simulink model "warplab_mimo_4x4"  (Simulink 6.6)
settings: Solver=ode45  StartTime=0.0  StopTime=50000  RelTol=1e-3
undefined symbols (not defined in the file): gcbh, xlBlockLoadCallback, xlGetSimulinkPeriod
libraries: xbsIndex_r4 x305, WARP_Blockset x16
(part 2 of 4)

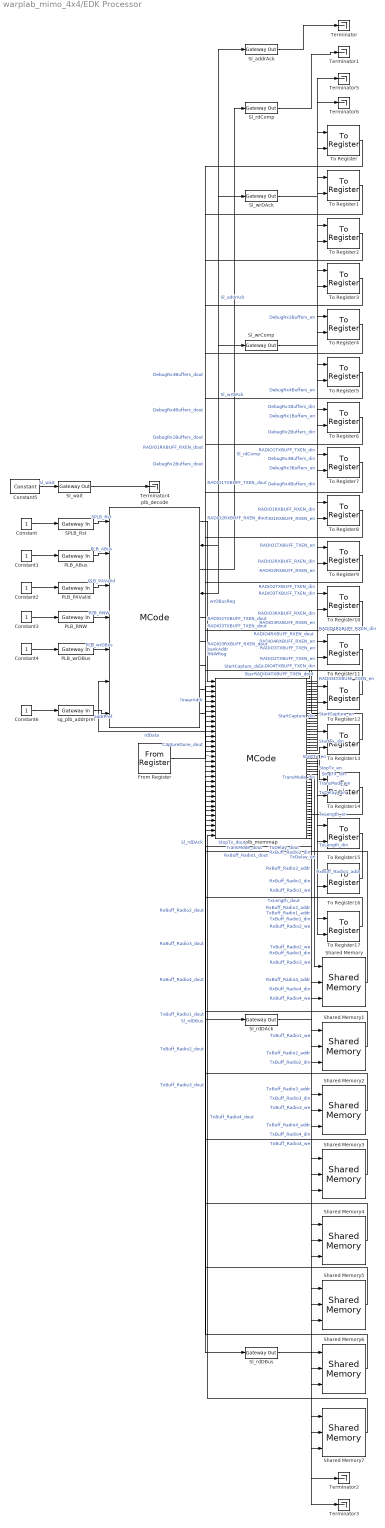
== system warplab_mimo_4x4/EDK Processor ==
  Constant{,1..4,6} (6 alike) : Constant
  Constant5 : xbsIndex_r4/Constant  arith_type=Unsigned  const=0  n_bits=1  bin_pt=0  explicit_period=on  period=xlGetSimulinkPeriod(gcb)  equ=P=C  opselect=C  inp2=PCIN>>17  opr=+  inp1=P  carry=CIN  dbl_ovrd=off  block_type=constant
  From Register : xbsIndex_r4/From Register  shared_memory_name='CaptureDone'  init=0  period=xlGetSimulinkPeriod(gcb)  ownership=Owned and initialized elsewhere  arith_type=Unsigned  n_bits=1  bin_pt=0  dbl_ovrd=off  block_type=fromreg
      settings: AttributesFormatString=<< %<shared_memory_name> >>  infoedit="Register block that reads data to a shared memory register.  Delay of one sample period."  block_version=10.1.3
  PLB_ABus : xbsIndex_r4/Gateway In  arith_type=Unsigned  n_bits=32  bin_pt=0  quantization="Round  (unbiased: +/- Inf)"  overflow=Saturate  period=xlGetSimulinkPeriod(gcb)  dbl_ovrd=off  timing_constraint=None  locs_specified=off  LOCs={}  block_type=gatewayin
      settings: infoedit="Gateway in block.  Converts inputs of type Simulink integer, double and fixed point to  Xilinx fixed point type.<P><P>Hardware notes:  In hardware these blocks become top level input ports."  sginterface={'Xilinx'=>{'jtaghwcosim'=>{'non_memory_mapped_port'=>'PLB_ABus'}},'iopad'=>{'constraint'=>'#'}}  block_version=10.1.3
  PLB_PAValid : xbsIndex_r4/Gateway In  arith_type=Unsigned  n_bits=1  bin_pt=0  quantization="Round  (unbiased: +/- Inf)"  overflow=Saturate  period=xlGetSimulinkPeriod(gcb)  dbl_ovrd=off  timing_constraint=None  locs_specified=off  LOCs={}  block_type=gatewayin
      settings: infoedit="Gateway in block.  Converts inputs of type Simulink integer, double and fixed point to  Xilinx fixed point type.<P><P>Hardware notes:  In hardware these blocks become top level input ports."  sginterface={'Xilinx'=>{'jtaghwcosim'=>{'non_memory_mapped_port'=>'PLB_PAValid'}},'iopad'=>{'constraint'=>'#'}}  block_version=10.1.3
  PLB_RNW : xbsIndex_r4/Gateway In  arith_type=Unsigned  n_bits=1  bin_pt=0  quantization="Round  (unbiased: +/- Inf)"  overflow=Saturate  period=xlGetSimulinkPeriod(gcb)  dbl_ovrd=off  timing_constraint=None  locs_specified=off  LOCs={}  block_type=gatewayin
      settings: infoedit="Gateway in block.  Converts inputs of type Simulink integer, double and fixed point to  Xilinx fixed point type.<P><P>Hardware notes:  In hardware these blocks become top level input ports."  sginterface={'Xilinx'=>{'jtaghwcosim'=>{'non_memory_mapped_port'=>'PLB_RNW'}},'iopad'=>{'constraint'=>'#'}}  block_version=10.1.3
  PLB_wrDBus : xbsIndex_r4/Gateway In  arith_type=Unsigned  n_bits=32  bin_pt=0  quantization="Round  (unbiased: +/- Inf)"  overflow=Saturate  period=xlGetSimulinkPeriod(gcb)  dbl_ovrd=off  timing_constraint=None  locs_specified=off  LOCs={}  block_type=gatewayin
      settings: infoedit="Gateway in block.  Converts inputs of type Simulink integer, double and fixed point to  Xilinx fixed point type.<P><P>Hardware notes:  In hardware these blocks become top level input ports."  sginterface={'Xilinx'=>{'jtaghwcosim'=>{'non_memory_mapped_port'=>'PLB_wrDBus'}},'iopad'=>{'constraint'=>'#'}}  block_version=10.1.3
  SPLB_Rst : xbsIndex_r4/Gateway In  arith_type=Unsigned  n_bits=1  bin_pt=0  quantization="Round  (unbiased: +/- Inf)"  overflow=Saturate  period=xlGetSimulinkPeriod(gcb)  dbl_ovrd=off  timing_constraint=None  locs_specified=off  LOCs={}  block_type=gatewayin
      settings: infoedit="Gateway in block.  Converts inputs of type Simulink integer, double and fixed point to  Xilinx fixed point type.<P><P>Hardware notes:  In hardware these blocks become top level input ports."  sginterface={'Xilinx'=>{'jtaghwcosim'=>{'non_memory_mapped_port'=>'SPLB_Rst'}},'iopad'=>{'constraint'=>'#'}}  block_version=10.1.3
  Shared Memory : xbsIndex_r4/Shared Memory  shared_memory_name='RxBuff_Radio1'  depth=16384  ownership=Owned and Initialized Elsewhere  initVector=sin(pi*(0:15)/16)  mutex=Unprotected  mode=Read and Write  write_mode=Read After Write  time_out=0  latency=1  explicit_data_type=off  arith_type=Unsigned  n_bits=32  bin_pt=0  implementation=Block RAM  use_rpm=off  block_type=shmem
      settings: AttributesFormatString=<< %<shared_memory_name> >>  block_version=10.1.3
  Shared Memory1 : xbsIndex_r4/Shared Memory  shared_memory_name='RxBuff_Radio2'  depth=16384  ownership=Owned and Initialized Elsewhere  initVector=sin(pi*(0:15)/16)  mutex=Unprotected  mode=Read and Write  write_mode=Read After Write  time_out=0  latency=1  explicit_data_type=off  arith_type=Unsigned  n_bits=32  bin_pt=0  implementation=Block RAM  use_rpm=off  block_type=shmem
      settings: AttributesFormatString=<< %<shared_memory_name> >>  block_version=10.1.3
  Shared Memory2 : xbsIndex_r4/Shared Memory  shared_memory_name='RxBuff_Radio3'  depth=16384  ownership=Owned and Initialized Elsewhere  initVector=sin(pi*(0:15)/16)  mutex=Unprotected  mode=Read and Write  write_mode=Read After Write  time_out=0  latency=1  explicit_data_type=off  arith_type=Unsigned  n_bits=32  bin_pt=0  implementation=Block RAM  use_rpm=off  block_type=shmem
      settings: AttributesFormatString=<< %<shared_memory_name> >>  block_version=10.1.3
  Shared Memory3 : xbsIndex_r4/Shared Memory  shared_memory_name='RxBuff_Radio4'  depth=16384  ownership=Owned and Initialized Elsewhere  initVector=sin(pi*(0:15)/16)  mutex=Unprotected  mode=Read and Write  write_mode=Read After Write  time_out=0  latency=1  explicit_data_type=off  arith_type=Unsigned  n_bits=32  bin_pt=0  implementation=Block RAM  use_rpm=off  block_type=shmem
      settings: AttributesFormatString=<< %<shared_memory_name> >>  block_version=10.1.3
  Shared Memory4 : xbsIndex_r4/Shared Memory  shared_memory_name='TxBuff_Radio1'  depth=16384  ownership=Owned and Initialized Elsewhere  initVector=sin(pi*(0:15)/16)  mutex=Unprotected  mode=Read and Write  write_mode=Read After Write  time_out=0  latency=1  explicit_data_type=off  arith_type=Unsigned  n_bits=32  bin_pt=0  implementation=Block RAM  use_rpm=off  block_type=shmem
      settings: AttributesFormatString=<< %<shared_memory_name> >>  block_version=10.1.3
  Shared Memory5 : xbsIndex_r4/Shared Memory  shared_memory_name='TxBuff_Radio2'  depth=16384  ownership=Owned and Initialized Elsewhere  initVector=sin(pi*(0:15)/16)  mutex=Unprotected  mode=Read and Write  write_mode=Read After Write  time_out=0  latency=1  explicit_data_type=off  arith_type=Unsigned  n_bits=32  bin_pt=0  implementation=Block RAM  use_rpm=off  block_type=shmem
      settings: AttributesFormatString=<< %<shared_memory_name> >>  block_version=10.1.3
  Shared Memory6 : xbsIndex_r4/Shared Memory  shared_memory_name='TxBuff_Radio3'  depth=16384  ownership=Owned and Initialized Elsewhere  initVector=sin(pi*(0:15)/16)  mutex=Unprotected  mode=Read and Write  write_mode=Read After Write  time_out=0  latency=1  explicit_data_type=off  arith_type=Unsigned  n_bits=32  bin_pt=0  implementation=Block RAM  use_rpm=off  block_type=shmem
      settings: AttributesFormatString=<< %<shared_memory_name> >>  block_version=10.1.3
  Shared Memory7 : xbsIndex_r4/Shared Memory  shared_memory_name='TxBuff_Radio4'  depth=16384  ownership=Owned and Initialized Elsewhere  initVector=sin(pi*(0:15)/16)  mutex=Unprotected  mode=Read and Write  write_mode=Read After Write  time_out=0  latency=1  explicit_data_type=off  arith_type=Unsigned  n_bits=32  bin_pt=0  implementation=Block RAM  use_rpm=off  block_type=shmem
      settings: AttributesFormatString=<< %<shared_memory_name> >>  block_version=10.1.3
  Sl_addrAck : xbsIndex_r4/Gateway Out  hdl_port=on  timing_constraint=None  locs_specified=off  LOCs={}  block_type=gatewayout
      settings: infoedit="Gateway out block.  Converts Xilinx fixed point inputs into ouputs of type Simulink integer, double, or fixed point.<P><P>Hardware notes:  In hardware these blocks become top level output ports or are discarded, depending on how they are configured."  sginterface={'Xilinx'=>{'jtaghwcosim'=>{'non_memory_mapped_port'=>'Sl_addrAck'}},'iopad'=>{'constraint'=>'#'}}  block_version=10.1.3
  Sl_rdComp : xbsIndex_r4/Gateway Out  hdl_port=on  timing_constraint=None  locs_specified=off  LOCs={}  block_type=gatewayout
      settings: infoedit="Gateway out block.  Converts Xilinx fixed point inputs into ouputs of type Simulink integer, double, or fixed point.<P><P>Hardware notes:  In hardware these blocks become top level output ports or are discarded, depending on how they are configured."  sginterface={'Xilinx'=>{'jtaghwcosim'=>{'non_memory_mapped_port'=>'Sl_rdComp'}},'iopad'=>{'constraint'=>'#'}}  block_version=10.1.3
  Sl_rdDAck : xbsIndex_r4/Gateway Out  hdl_port=on  timing_constraint=None  locs_specified=off  LOCs={}  block_type=gatewayout
      settings: infoedit="Gateway out block.  Converts Xilinx fixed point inputs into ouputs of type Simulink integer, double, or fixed point.<P><P>Hardware notes:  In hardware these blocks become top level output ports or are discarded, depending on how they are configured."  sginterface={'Xilinx'=>{'jtaghwcosim'=>{'non_memory_mapped_port'=>'Sl_rdDAck'}},'iopad'=>{'constraint'=>'#'}}  block_version=10.1.3
  Sl_rdDBus : xbsIndex_r4/Gateway Out  hdl_port=on  timing_constraint=None  locs_specified=off  LOCs={}  block_type=gatewayout
      settings: infoedit="Gateway out block.  Converts Xilinx fixed point inputs into ouputs of type Simulink integer, double, or fixed point.<P><P>Hardware notes:  In hardware these blocks become top level output ports or are discarded, depending on how they are configured."  sginterface={'Xilinx'=>{'jtaghwcosim'=>{'non_memory_mapped_port'=>'Sl_rdDBus'}},'iopad'=>{'constraint'=>'#'}}  block_version=10.1.3
  Sl_wait : xbsIndex_r4/Gateway Out  hdl_port=on  timing_constraint=None  locs_specified=off  LOCs={}  block_type=gatewayout
      settings: infoedit="Gateway out block.  Converts Xilinx fixed point inputs into ouputs of type Simulink integer, double, or fixed point.<P><P>Hardware notes:  In hardware these blocks become top level output ports or are discarded, depending on how they are configured."  sginterface={'Xilinx'=>{'jtaghwcosim'=>{'non_memory_mapped_port'=>'Sl_wait'}},'iopad'=>{'constraint'=>'#'}}  block_version=10.1.3
  Sl_wrComp : xbsIndex_r4/Gateway Out  hdl_port=on  timing_constraint=None  locs_specified=off  LOCs={}  block_type=gatewayout
      settings: infoedit="Gateway out block.  Converts Xilinx fixed point inputs into ouputs of type Simulink integer, double, or fixed point.<P><P>Hardware notes:  In hardware these blocks become top level output ports or are discarded, depending on how they are configured."  sginterface={'Xilinx'=>{'jtaghwcosim'=>{'non_memory_mapped_port'=>'Sl_wrComp'}},'iopad'=>{'constraint'=>'#'}}  block_version=10.1.3
  Sl_wrDAck : xbsIndex_r4/Gateway Out  hdl_port=on  timing_constraint=None  locs_specified=off  LOCs={}  block_type=gatewayout
      settings: infoedit="Gateway out block.  Converts Xilinx fixed point inputs into ouputs of type Simulink integer, double, or fixed point.<P><P>Hardware notes:  In hardware these blocks become top level output ports or are discarded, depending on how they are configured."  sginterface={'Xilinx'=>{'jtaghwcosim'=>{'non_memory_mapped_port'=>'Sl_wrDAck'}},'iopad'=>{'constraint'=>'#'}}  block_version=10.1.3
  Terminator{,1..6} (7 alike) : Terminator
  To Register : xbsIndex_r4/To Register  shared_memory_name='DebugRx1Buffers'  init=0  ownership=Owned and initialized elsewhere  explicit_data_type=on  arith_type=Unsigned  n_bits=1  bin_pt=0  dbl_ovrd=off  block_type=toreg
      settings: AttributesFormatString=<< %<shared_memory_name> >>  infoedit="Register block that writes data to a shared memory register.  Delay of one sample period."  block_version=10.1.3
  To Register1 : xbsIndex_r4/To Register  shared_memory_name='DebugRx2Buffers'  init=0  ownership=Owned and initialized elsewhere  explicit_data_type=on  arith_type=Unsigned  n_bits=1  bin_pt=0  dbl_ovrd=off  block_type=toreg
      settings: AttributesFormatString=<< %<shared_memory_name> >>  infoedit="Register block that writes data to a shared memory register.  Delay of one sample period."  block_version=10.1.3
  To Register10 : xbsIndex_r4/To Register  shared_memory_name='RADIO4RXBUFF_RXEN'  init=0  ownership=Owned and initialized elsewhere  explicit_data_type=on  arith_type=Unsigned  n_bits=1  bin_pt=0  dbl_ovrd=off  block_type=toreg
      settings: AttributesFormatString=<< %<shared_memory_name> >>  infoedit="Register block that writes data to a shared memory register.  Delay of one sample period."  block_version=10.1.3
  To Register11 : xbsIndex_r4/To Register  shared_memory_name='RADIO4TXBUFF_TXEN'  init=0  ownership=Owned and initialized elsewhere  explicit_data_type=on  arith_type=Unsigned  n_bits=1  bin_pt=0  dbl_ovrd=off  block_type=toreg
      settings: AttributesFormatString=<< %<shared_memory_name> >>  infoedit="Register block that writes data to a shared memory register.  Delay of one sample period."  block_version=10.1.3
  To Register12 : xbsIndex_r4/To Register  shared_memory_name='StartCapture'  init=0  ownership=Owned and initialized elsewhere  explicit_data_type=on  arith_type=Unsigned  n_bits=1  bin_pt=0  dbl_ovrd=off  block_type=toreg
      settings: AttributesFormatString=<< %<shared_memory_name> >>  infoedit="Register block that writes data to a shared memory register.  Delay of one sample period."  block_version=10.1.3
  To Register13 : xbsIndex_r4/To Register  shared_memory_name='StartTx'  init=0  ownership=Owned and initialized elsewhere  explicit_data_type=on  arith_type=Unsigned  n_bits=1  bin_pt=0  dbl_ovrd=off  block_type=toreg
      settings: AttributesFormatString=<< %<shared_memory_name> >>  infoedit="Register block that writes data to a shared memory register.  Delay of one sample period."  block_version=10.1.3
  To Register14 : xbsIndex_r4/To Register  shared_memory_name='StopTx'  init=0  ownership=Owned and initialized elsewhere  explicit_data_type=on  arith_type=Unsigned  n_bits=1  bin_pt=0  dbl_ovrd=off  block_type=toreg
      settings: AttributesFormatString=<< %<shared_memory_name> >>  infoedit="Register block that writes data to a shared memory register.  Delay of one sample period."  block_version=10.1.3
  To Register15 : xbsIndex_r4/To Register  shared_memory_name='TransMode'  init=0  ownership=Owned and initialized elsewhere  explicit_data_type=on  arith_type=Unsigned  n_bits=1  bin_pt=0  dbl_ovrd=off  block_type=toreg
      settings: AttributesFormatString=<< %<shared_memory_name> >>  infoedit="Register block that writes data to a shared memory register.  Delay of one sample period."  block_version=10.1.3
  To Register16 : xbsIndex_r4/To Register  shared_memory_name='TxDelay'  init=0  ownership=Owned and initialized elsewhere  explicit_data_type=on  arith_type=Unsigned  n_bits=14  bin_pt=0  dbl_ovrd=off  block_type=toreg
      settings: AttributesFormatString=<< %<shared_memory_name> >>  infoedit="Register block that writes data to a shared memory register.  Delay of one sample period."  block_version=10.1.3
  To Register17 : xbsIndex_r4/To Register  shared_memory_name='TxLength'  init=0  ownership=Owned and initialized elsewhere  explicit_data_type=on  arith_type=Unsigned  n_bits=14  bin_pt=0  dbl_ovrd=off  block_type=toreg
      settings: AttributesFormatString=<< %<shared_memory_name> >>  infoedit="Register block that writes data to a shared memory register.  Delay of one sample period."  block_version=10.1.3
  To Register2 : xbsIndex_r4/To Register  shared_memory_name='DebugRx3Buffers'  init=0  ownership=Owned and initialized elsewhere  explicit_data_type=on  arith_type=Unsigned  n_bits=1  bin_pt=0  dbl_ovrd=off  block_type=toreg
      settings: AttributesFormatString=<< %<shared_memory_name> >>  infoedit="Register block that writes data to a shared memory register.  Delay of one sample period."  block_version=10.1.3
  To Register3 : xbsIndex_r4/To Register  shared_memory_name='DebugRx4Buffers'  init=0  ownership=Owned and initialized elsewhere  explicit_data_type=on  arith_type=Unsigned  n_bits=1  bin_pt=0  dbl_ovrd=off  block_type=toreg
      settings: AttributesFormatString=<< %<shared_memory_name> >>  infoedit="Register block that writes data to a shared memory register.  Delay of one sample period."  block_version=10.1.3
  To Register4 : xbsIndex_r4/To Register  shared_memory_name='RADIO1RXBUFF_RXEN'  init=0  ownership=Owned and initialized elsewhere  explicit_data_type=on  arith_type=Unsigned  n_bits=1  bin_pt=0  dbl_ovrd=off  block_type=toreg
      settings: AttributesFormatString=<< %<shared_memory_name> >>  infoedit="Register block that writes data to a shared memory register.  Delay of one sample period."  block_version=10.1.3
  To Register5 : xbsIndex_r4/To Register  shared_memory_name='RADIO1TXBUFF_TXEN'  init=0  ownership=Owned and initialized elsewhere  explicit_data_type=on  arith_type=Unsigned  n_bits=1  bin_pt=0  dbl_ovrd=off  block_type=toreg
      settings: AttributesFormatString=<< %<shared_memory_name> >>  infoedit="Register block that writes data to a shared memory register.  Delay of one sample period."  block_version=10.1.3
  To Register6 : xbsIndex_r4/To Register  shared_memory_name='RADIO2RXBUFF_RXEN'  init=0  ownership=Owned and initialized elsewhere  explicit_data_type=on  arith_type=Unsigned  n_bits=1  bin_pt=0  dbl_ovrd=off  block_type=toreg
      settings: AttributesFormatString=<< %<shared_memory_name> >>  infoedit="Register block that writes data to a shared memory register.  Delay of one sample period."  block_version=10.1.3
  To Register7 : xbsIndex_r4/To Register  shared_memory_name='RADIO2TXBUFF_TXEN'  init=0  ownership=Owned and initialized elsewhere  explicit_data_type=on  arith_type=Unsigned  n_bits=1  bin_pt=0  dbl_ovrd=off  block_type=toreg
      settings: AttributesFormatString=<< %<shared_memory_name> >>  infoedit="Register block that writes data to a shared memory register.  Delay of one sample period."  block_version=10.1.3
  To Register8 : xbsIndex_r4/To Register  shared_memory_name='RADIO3RXBUFF_RXEN'  init=0  ownership=Owned and initialized elsewhere  explicit_data_type=on  arith_type=Unsigned  n_bits=1  bin_pt=0  dbl_ovrd=off  block_type=toreg
      settings: AttributesFormatString=<< %<shared_memory_name> >>  infoedit="Register block that writes data to a shared memory register.  Delay of one sample period."  block_version=10.1.3
  To Register9 : xbsIndex_r4/To Register  shared_memory_name='RADIO3TXBUFF_TXEN'  init=0  ownership=Owned and initialized elsewhere  explicit_data_type=on  arith_type=Unsigned  n_bits=1  bin_pt=0  dbl_ovrd=off  block_type=toreg
      settings: AttributesFormatString=<< %<shared_memory_name> >>  infoedit="Register block that writes data to a shared memory register.  Delay of one sample period."  block_version=10.1.3
  plb_decode : xbsIndex_r4/MCode  mfname=xlmax  explicit_period=off  period=1  dbl_ovrd=off  enable_stdout=off  enable_debug=off  mfilecontent=|  suppress_output=1  defparams={}  hide_port_list={}  block_type=mcode
      | function [wrDBusReg, addrAck, rdComp, wrDAck, bankAddr, RNWReg, rdDAck, rdDBus, linearAddr] = ...
      |     plb_bus_decode(plbRst, plbABus, plbPAValid, plbRNW, plbWrDBus, rdData, addrPref)
      | 
      | % constant variables (TODO: should pass from outside)
      | ADDRPREF_LEN = 11;
      | BANKADDR_LEN = 2;
      | LINEARADDR_LEN = 17;
      | ABUS_LEN = 32;
      | DBUS_LEN = 32;
      | 
      | % declare and initialize persistent variables
      | % register input bus signals
      | persistent plbRstReg_, plbRstReg_ = xl_state(0, {xlBoolean});
      | persistent plbABusReg_, plbABusReg_ = xl_state(0, {xlUnsigned, ABUS_LEN, 0});
      | persistent plbPAValidReg_, plbPAValidReg_ = xl_state(0, {xlBoolean});
      | persistent plbRNWReg_, plbRNWReg_ = xl_state(0, {xlUnsigned, 1, 0});
      | persistent plbWrDBusReg_, plbWrDBusReg_ = xl_state(0, {xlUnsigned, DBUS_LEN, 0});
      | 
      | % ===== rest of the outputs =====
      | 
      | bankAddr   = xl_slice(plbABusReg_, 2+BANKADDR_LEN+LINEARADDR_LEN-1, 2+LINEARADDR_LEN);
      | linearAddr = xl_slice(plbABusReg_, 2+LINEARADDR_LEN-1, 2);
      | RNWReg = plbRNWReg_;
      | wrDBusReg = plbWrDBusReg_;
      | 
      | % ===== p_select =====
      | 
      | % register PAValid
      | persistent aValidReg, aValidReg = xl_state(0, {xlBoolean});
      | aValidReg = plbPAValidReg_;
      | 
      | % extract and register the address prefix
      | addrPref_in = xl_slice(plbABusReg_, xl_nbits(plbABusReg_)-1, xl_nbits(plbABusReg_)-ADDRPREF_LEN);
      | if addrPref_in == addrPref
      |     ps1 = true;
      | else 
      |     ps1 = false;
      | end 
      | 
      | persistent ps1Reg, ps1Reg = xl_state(0, ps1);
      | ps1Reg = ps1;
      | 
      | ps = xl_and(ps1Reg, aValidReg);
      | 
      | % ===== addrAck =====
      | 
      | % register ps
      | persistent psReg, psReg = xl_state(0, ps);
      | 
      | addrAck = xfix({xlUnsigned, 1, 0}, xl_and(xl_not(plbRstReg_), ps, xl_not(psReg)));
      | 
      | psReg = ps;
      | 
      | % ===== rdComp, rd/wr DAck =====
      |  
      | rdComp1 = xfix({xlUnsigned, 1, 0}, xl_and(addrAck, RNWReg));
      | 
      | NUM_rdCompDelay = 3;
      | persistent rdCompDelay, rdCompDelay = xl_state(zeros(1, NUM_rdCompDelay), rdComp1, NUM_rdCompDelay);
      | rdComp2 = rdCompDelay.back;
      | rdCompDelay.push_front_pop_back(rdComp1);
      | 
      | persistent rdCompReg, rdCompReg = xl_state(0, rdComp1);
      | rdComp = rdCompReg;
      | rdCompReg = rdComp2;
      | 
      | persistent rdDAckReg, rdDAckReg = xl_state(0, rdComp1);
      | rdDAck = rdDAckReg;
      | rdDAckReg = rdComp;
      | 
      | persistent wrDAckReg, wrDAckReg = xl_state(0, addrAck);
      | wrDAck = wrDAckReg;
      | wrDAckReg = xl_and(addrAck, xl_not(RNWReg));
      | 
      | % ===== rdDBus =====
      | 
      | rdSel = xl_or(rdComp2, rdComp);
      | 
      | if rdSel == 1
      |     rdDBus1 = rdData;
      | else
      |     rdDBus1 = 0;
      | end % if
      | 
      | persistent rdDBusReg, rdDBusReg = xl_state(0, rdDBus1);
      | rdDBus = rdDBusReg;
      | rdDBusReg = rdDBus1;
      | 
      | % rdDBus = xl_concat(rdDBus32, rdDBus32);
      | % rdDBus = rdDBus32;
      | 
      | % ===== update the persistent variables =====
      | 
      | plbRstReg_ = plbRst;
      | plbABusReg_ = plbABus;
      | plbPAValidReg_ = plbPAValid;
      | plbRNWReg_ = plbRNW;
      | plbWrDBusReg_ = xl_slice(plbWrDBus, DBUS_LEN-1, 0);
      settings: block_version=10.1.3
  plb_memmap : xbsIndex_r4/MCode  mfname=xlmax  explicit_period=off  period=1  dbl_ovrd=off  enable_stdout=off  enable_debug=off  mfilecontent=|  suppress_output=1  defparams={}  hide_port_list={}  block_type=mcode
      | function [read_bank_out, sm_DebugRx1Buffers_din, sm_DebugRx1Buffers_en, sm_DebugRx2Buffers_din, sm_DebugRx2Buffers_en, sm_DebugRx3Buffers_din, sm_DebugRx3Buffers_en, sm_DebugRx4Buffers_din, sm_DebugRx4Buffers_en, sm_RADIO1RXBUFF_RXEN_din, sm_RADIO1RXBUFF_RXEN_en, sm_RADIO1TXBUFF_TXEN_din, sm_RADIO1TXBUFF_TXEN_en, sm_RADIO2RXBUFF_RXEN_din, sm_RADIO2RXBUFF_RXEN_en, sm_RADIO2TXBUFF_TXEN_din, sm_RADIO2TXBUFF_TXEN_en, sm_RADIO3RXBUFF_RXEN_din, sm_RADIO3RXBUFF_RXEN_en, sm_RADIO3TXBUFF_TXEN_din, sm_RADIO3TXBUFF_TXEN_en, sm_RADIO4RXBUFF_RXEN_din, sm_RADIO4RXBUFF_RXEN_en, sm_RADIO4TXBUFF_TXEN_din, sm_RADIO4TXBUFF_TXEN_en, sm_StartCapture_din, sm_StartCapture_en, sm_StartTx_din, sm_StartTx_en, sm_StopTx_din, sm_StopTx_en, sm_TransMode_din, sm_TransMode_en, sm_TxDelay_din, sm_TxDelay_en, sm_TxLength_din, sm_TxLength_en, sm_RxBuff_Radio1_addr, sm_RxBuff_Radio1_din, sm_RxBuff_Radio1_we, sm_RxBuff_Radio2_addr, sm_RxBuff_Radio2_din, sm_RxBuff_Radio2_we, sm_RxBuff_Radio3_addr, sm_RxBuff_Radio3_din, sm_RxBuff_Radio3_we, sm_RxBuff_Radio4_addr, sm_RxBuff_Radio4_din, sm_RxBuff_Radio4_we, sm_TxBuff_Radio1_addr, sm_TxBuff_Radio1_din, sm_TxBuff_Radio1_we, sm_TxBuff_Radio2_addr, sm_TxBuff_Radio2_din, sm_TxBuff_Radio2_we, sm_TxBuff_Radio3_addr, sm_TxBuff_Radio3_din, sm_TxBuff_Radio3_we, sm_TxBuff_Radio4_addr, sm_TxBuff_Radio4_din, sm_TxBuff_Radio4_we] = plb_memmap(wrDBus, bankAddr, linearAddr, RNWReg, addrAck, sm_CaptureDone, sm_DebugRx1Buffers, sm_DebugRx2Buffers, sm_DebugRx3Buffers, sm_DebugRx4Buffers, sm_RADIO1RXBUFF_RXEN, sm_RADIO1TXBUFF_TXEN, sm_RADIO2RXBUFF_RXEN, sm_RADIO2TXBUFF_TXEN, sm_RADIO3RXBUFF_RXEN, sm_RADIO3TXBUFF_TXEN, sm_RADIO4RXBUFF_RXEN, sm_RADIO4TXBUFF_TXEN, sm_StartCapture, sm_StartTx, sm_StopTx, sm_TransMode, sm_TxDelay, sm_TxLength, sm_RxBuff_Radio1, sm_RxBuff_Radio2, sm_RxBuff_Radio3, sm_RxBuff_Radio4, sm_TxBuff_Radio1, sm_TxBuff_Radio2, sm_TxBuff_Radio3, sm_TxBuff_Radio4)
      | 
      | 
      | % connvert the input data to UFix_32_0 (the bus data type)
      | % 'From Register' blocks
      | % sm_CaptureDone_bus = xfix({xlUnsigned, 32, 0}, 0);
      | sm_CaptureDone_bus = xl_force(sm_CaptureDone, xlUnsigned, 0);
      | 
      | % 'To Register' blocks
      | 
      | % sm_DebugRx1Buffers_dout = xfix({xlUnsigned, 32, 0}, 0);
      | sm_DebugRx1Buffers_dout = xl_force(sm_DebugRx1Buffers, xlUnsigned, 0);
      | 
      | % sm_DebugRx2Buffers_dout = xfix({xlUnsigned, 32, 0}, 0);
      | sm_DebugRx2Buffers_dout = xl_force(sm_DebugRx2Buffers, xlUnsigned, 0);
      | 
      | % sm_DebugRx3Buffers_dout = xfix({xlUnsigned, 32, 0}, 0);
      | sm_DebugRx3Buffers_dout = xl_force(sm_DebugRx3Buffers, xlUnsigned, 0);
      | 
      | % sm_DebugRx4Buffers_dout = xfix({xlUnsigned, 32, 0}, 0);
      | sm_DebugRx4Buffers_dout = xl_force(sm_DebugRx4Buffers, xlUnsigned, 0);
      | 
      | % sm_RADIO1RXBUFF_RXEN_dout = xfix({xlUnsigned, 32, 0}, 0);
      | sm_RADIO1RXBUFF_RXEN_dout = xl_force(sm_RADIO1RXBUFF_RXEN, xlUnsigned, 0);
      | 
      | % sm_RADIO1TXBUFF_TXEN_dout = xfix({xlUnsigned, 32, 0}, 0);
      | sm_RADIO1TXBUFF_TXEN_dout = xl_force(sm_RADIO1TXBUFF_TXEN, xlUnsigned, 0);
      | 
      | % sm_RADIO2RXBUFF_RXEN_dout = xfix({xlUnsigned, 32, 0}, 0);
      | sm_RADIO2RXBUFF_RXEN_dout = xl_force(sm_RADIO2RXBUFF_RXEN, xlUnsigned, 0);
      | 
      | % sm_RADIO2TXBUFF_TXEN_dout = xfix({xlUnsigned, 32, 0}, 0);
      | sm_RADIO2TXBUFF_TXEN_dout = xl_force(sm_RADIO2TXBUFF_TXEN, xlUnsigned, 0);
      | 
      | % sm_RADIO3RXBUFF_RXEN_dout = xfix({xlUnsigned, 32, 0}, 0);
      | sm_RADIO3RXBUFF_RXEN_dout = xl_force(sm_RADIO3RXBUFF_RXEN, xlUnsigned, 0);
      | 
      | % sm_RADIO3TXBUFF_TXEN_dout = xfix({xlUnsigned, 32, 0}, 0);
      | sm_RADIO3TXBUFF_TXEN_dout = xl_force(sm_RADIO3TXBUFF_TXEN, xlUnsigned, 0);
      | 
      | % sm_RADIO4RXBUFF_RXEN_dout = xfix({xlUnsigned, 32, 0}, 0);
      | sm_RADIO4RXBUFF_RXEN_dout = xl_force(sm_RADIO4RXBUFF_RXEN, xlUnsigned, 0);
      | 
      | % sm_RADIO4TXBUFF_TXEN_dout = xfix({xlUnsigned, 32, 0}, 0);
      | sm_RADIO4TXBUFF_TXEN_dout = xl_force(sm_RADIO4TXBUFF_TXEN, xlUnsigned, 0);
      | 
      | % sm_StartCapture_dout = xfix({xlUnsigned, 32, 0}, 0);
      | sm_StartCapture_dout = xl_force(sm_StartCapture, xlUnsigned, 0);
      | 
      | % sm_StartTx_dout = xfix({xlUnsigned, 32, 0}, 0);
      | sm_StartTx_dout = xl_force(sm_StartTx, xlUnsigned, 0);
      | 
      | % sm_StopTx_dout = xfix({xlUnsigned, 32, 0}, 0);
      | sm_StopTx_dout = xl_force(sm_StopTx, xlUnsigned, 0);
      | 
      | % sm_TransMode_dout = xfix({xlUnsigned, 32, 0}, 0);
      | sm_TransMode_dout = xl_force(sm_TransMode, xlUnsigned, 0);
      | 
      | % sm_TxDelay_dout = xfix({xlUnsigned, 32, 0}, 0);
      | sm_TxDelay_dout = xl_force(sm_TxDelay, xlUnsigned, 0);
      | 
      | % sm_TxLength_dout = xfix({xlUnsigned, 32, 0}, 0);
      | sm_TxLength_dout = xl_force(sm_TxLength, xlUnsigned, 0);
      | 
      | 
      | % 'From FIFO' blocks
      | % 'To FIFO' blocks
      | % 'Shared Memory' blocks
      | % RxBuff_Radio1_bus = xfix({xlUnsigned, 32, 0}, 0);
      | sm_RxBuff_Radio1_bus = xl_force(sm_RxBuff_Radio1, xlUnsigned, 0);
      | 
      | % RxBuff_Radio2_bus = xfix({xlUnsigned, 32, 0}, 0);
      | sm_RxBuff_Radio2_bus = xl_force(sm_RxBuff_Radio2, xlUnsigned, 0);
      | 
      | % RxBuff_Radio3_bus = xfix({xlUnsigned, 32, 0}, 0);
      | sm_RxBuff_Radio3_bus = xl_force(sm_RxBuff_Radio3, xlUnsigned, 0);
      | 
      | % RxBuff_Radio4_bus = xfix({xlUnsigned, 32, 0}, 0);
      | sm_RxBuff_Radio4_bus = xl_force(sm_RxBuff_Radio4, xlUnsigned, 0);
      | 
      | % TxBuff_Radio1_bus = xfix({xlUnsigned, 32, 0}, 0);
      | sm_TxBuff_Radio1_bus = xl_force(sm_TxBuff_Radio1, xlUnsigned, 0);
      | 
      | % TxBuff_Radio2_bus = xfix({xlUnsigned, 32, 0}, 0);
      | sm_TxBuff_Radio2_bus = xl_force(sm_TxBuff_Radio2, xlUnsigned, 0);
      | 
      | % TxBuff_Radio3_bus = xfix({xlUnsigned, 32, 0}, 0);
      | sm_TxBuff_Radio3_bus = xl_force(sm_TxBuff_Radio3, xlUnsigned, 0);
      | 
      | % TxBuff_Radio4_bus = xfix({xlUnsigned, 32, 0}, 0);
      | sm_TxBuff_Radio4_bus = xl_force(sm_TxBuff_Radio4, xlUnsigned, 0);
      | 
      | 
      | % 'dout' ports of 'From Register' blocks
      | 
      | % registered register mux output
      | persistent reg_bank_out_reg; reg_bank_out_reg = xl_state(0, {xlUnsigned, 32, 0});
      | reg_bank_out = reg_bank_out_reg;
      | 
      | if linearAddr == 18
      |     reg_bank_out_reg = sm_CaptureDone_bus;
      | elseif linearAddr == 0
      |     reg_bank_out_reg = sm_DebugRx1Buffers_dout;
      | elseif linearAddr == 1
      |     reg_bank_out_reg = sm_DebugRx2Buffers_dout;
      | elseif linearAddr == 2
      |     reg_bank_out_reg = sm_DebugRx3Buffers_dout;
      | elseif linearAddr == 3
      |     reg_bank_out_reg = sm_DebugRx4Buffers_dout;
      | elseif linearAddr == 4
      |     reg_bank_out_reg = sm_RADIO1RXBUFF_RXEN_dout;
      | elseif linearAddr == 5
      |     reg_bank_out_reg = sm_RADIO1TXBUFF_TXEN_dout;
      | elseif linearAddr == 6
      |     reg_bank_out_reg = sm_RADIO2RXBUFF_RXEN_dout;
      | elseif linearAddr == 7
      |     reg_bank_out_reg = sm_RADIO2TXBUFF_TXEN_dout;
      | elseif linearAddr == 8
      |     reg_bank_out_reg = sm_RADIO3RXBUFF_RXEN_dout;
      | elseif linearAddr == 9
      |     reg_bank_out_reg = sm_RADIO3TXBUFF_TXEN_dout;
      | elseif linearAddr == 10
      |     reg_bank_out_reg = sm_RADIO4RXBUFF_RXEN_dout;
      | elseif linearAddr == 11
      |     reg_bank_out_reg = sm_RADIO4TXBUFF_TXEN_dout;
      | elseif linearAddr == 12
      |     reg_bank_out_reg = sm_StartCapture_dout;
      | elseif linearAddr == 13
      |     reg_bank_out_reg = sm_StartTx_dout;
      | elseif linearAddr == 14
      |     reg_bank_out_reg = sm_StopTx_dout;
      | elseif linearAddr == 15
      |     reg_bank_out_reg = sm_TransMode_dout;
      | elseif linearAddr == 16
      |     reg_bank_out_reg = sm_TxDelay_dout;
      | elseif linearAddr == 17
      |     reg_bank_out_reg = sm_TxLength_dout;
      | 
      | end
      | 
      | 
      | % 'From FIFO' and 'To FIFO' blocks
      | 
      | 
      | 
      | 
      | 
      | opCode = xl_concat(addrAck, RNWReg, bankAddr, linearAddr);
      | 
      | % 'Shared Memory' blocks
      | 
      | sm_RxBuff_Radio1_sel_value = xl_concat(xl_slice(linearAddr, ...
      |                                         xl_nbits(linearAddr) - 1, ...
      |                                         14) ...
      |                                     );
      | if sm_RxBuff_Radio1_sel_value == xfix({xlUnsigned, ...
      |                                         xl_nbits(linearAddr) - 14, ...
      |                                         0}, ...
      |                                         0);
      |     sm_RxBuff_Radio1_sel = true;
      | else
      |     sm_RxBuff_Radio1_sel = false;
      | end
      | sm_RxBuff_Radio2_sel_value = xl_concat(xl_slice(linearAddr, ...
      |                                         xl_nbits(linearAddr) - 1, ...
      |                                         14) ...
      |                                     );
      | if sm_RxBuff_Radio2_sel_value == xfix({xlUnsigned, ...
      |                                         xl_nbits(linearAddr) - 14, ...
      |                                         0}, ...
      |                                         1);
      |     sm_RxBuff_Radio2_sel = true;
      | else
      |     sm_RxBuff_Radio2_sel = false;
      | end
      | sm_RxBuff_Radio3_sel_value = xl_concat(xl_slice(linearAddr, ...
      |                                         xl_nbits(linearAddr) - 1, ...
      |                                         14) ...
      |                                     );
      | if sm_RxBuff_Radio3_sel_value == xfix({xlUnsigned, ...
      |                                         xl_nbits(linearAddr) - 14, ...
      |                                         0}, ...
      |                                         2);
      |     sm_RxBuff_Radio3_sel = true;
      | else
      |     sm_RxBuff_Radio3_sel = false;
      | end
      | sm_RxBuff_Radio4_sel_value = xl_concat(xl_slice(linearAddr, ...
      |                                         xl_nbits(linearAddr) - 1, ...
      |                                         14) ...
      |                                     );
      | if sm_RxBuff_Radio4_sel_value == xfix({xlUnsigned, ...
      |                                         xl_nbits(linearAddr) - 14, ...
      |                                         0}, ...
      |                                         3);
      |     sm_RxBuff_Radio4_sel = true;
      | else
      |     sm_RxBuff_Radio4_sel = false;
      | end
      | sm_TxBuff_Radio1_sel_value = xl_concat(xl_slice(linearAddr, ...
      |                                         xl_nbits(linearAddr) - 1, ...
      |                                         14) ...
      |                                     );
      | if sm_TxBuff_Radio1_sel_value == xfix({xlUnsigned, ...
      |                                         xl_nbits(linearAddr) - 14, ...
      |                                         0}, ...
      |                                         4);
      |     sm_TxBuff_Radio1_sel = true;
      | else
      |     sm_TxBuff_Radio1_sel = false;
      | end
      | sm_TxBuff_Radio2_sel_value = xl_concat(xl_slice(linearAddr, ...
      |                                         xl_nbits(linearAddr) - 1, ...
      |                                         14) ...
      |                                     );
      | if sm_TxBuff_Radio2_sel_value == xfix({xlUnsigned, ...
      |                                         xl_nbits(linearAddr) - 14, ...
      |                                         0}, ...
      |                                         5);
      |     sm_TxBuff_Radio2_sel = true;
      | else
      |     sm_TxBuff_Radio2_sel = false;
      | end
      | sm_TxBuff_Radio3_sel_value = xl_concat(xl_slice(linearAddr, ...
      |                                         xl_nbits(linearAddr) - 1, ...
      |                                         14) ...
      |                                     );
      | if sm_TxBuff_Radio3_sel_value == xfix({xlUnsigned, ...
      |                                         xl_nbits(linearAddr) - 14, ...
      |                                         0}, ...
      |                                         6);
      |     sm_TxBuff_Radio3_sel = true;
      | else
      |     sm_TxBuff_Radio3_sel = false;
      | end
      | sm_TxBuff_Radio4_sel_value = xl_concat(xl_slice(linearAddr, ...
      |                                         xl_nbits(linearAddr) - 1, ...
      |                                         14) ...
      |                                     );
      | if sm_TxBuff_Radio4_sel_value == xfix({xlUnsigned, ...
      |                                         xl_nbits(linearAddr) - 14, ...
      |                                         0}, ...
      |                                         7);
      |     sm_TxBuff_Radio4_sel = true;
      | else
      |     sm_TxBuff_Radio4_sel = false;
      | end
      | 
      | 
      | % registered Shared Memory mux output
      | persistent ram_bank_out_reg; ram_bank_out_reg = xl_state(0, {xlUnsigned, 32, 0});
      | ram_bank_out = ram_bank_out_reg;
      | if sm_RxBuff_Radio1_sel
      |     ram_bank_out_reg = sm_RxBuff_Radio1_bus;
      | elseif sm_RxBuff_Radio2_sel
      |     ram_bank_out_reg = sm_RxBuff_Radio2_bus;
      | elseif sm_RxBuff_Radio3_sel
      |     ram_bank_out_reg = sm_RxBuff_Radio3_bus;
      | elseif sm_RxBuff_Radio4_sel
      |     ram_bank_out_reg = sm_RxBuff_Radio4_bus;
      | elseif sm_TxBuff_Radio1_sel
      |     ram_bank_out_reg = sm_TxBuff_Radio1_bus;
      | elseif sm_TxBuff_Radio2_sel
      |     ram_bank_out_reg = sm_TxBuff_Radio2_bus;
      | elseif sm_TxBuff_Radio3_sel
      |     ram_bank_out_reg = sm_TxBuff_Radio3_bus;
      | elseif sm_TxBuff_Radio4_sel
      |     ram_bank_out_reg = sm_TxBuff_Radio4_bus;
      | end
      | 
      | % 'din' ports of 'Shared Memory' blocks
      | sm_RxBuff_Radio1_din = xl_force(xl_slice(wrDBus, 32 - 1, 0), ...
      |                                  xlUnsigned, ...
      |                                  0);
      | sm_RxBuff_Radio2_din = xl_force(xl_slice(wrDBus, 32 - 1, 0), ...
      |                                  xlUnsigned, ...
      |                                  0);
      | sm_RxBuff_Radio3_din = xl_force(xl_slice(wrDBus, 32 - 1, 0), ...
      |                                  xlUnsigned, ...
      |                                  0);
      | sm_RxBuff_Radio4_din = xl_force(xl_slice(wrDBus, 32 - 1, 0), ...
      |                                  xlUnsigned, ...
      |                                  0);
      | sm_TxBuff_Radio1_din = xl_force(xl_slice(wrDBus, 32 - 1, 0), ...
      |                                  xlUnsigned, ...
      |                                  0);
      | sm_TxBuff_Radio2_din = xl_force(xl_slice(wrDBus, 32 - 1, 0), ...
      |                                  xlUnsigned, ...
      |                                  0);
      | sm_TxBuff_Radio3_din = xl_force(xl_slice(wrDBus, 32 - 1, 0), ...
      |                                  xlUnsigned, ...
      |                                  0);
      | sm_TxBuff_Radio4_din = xl_force(xl_slice(wrDBus, 32 - 1, 0), ...
      |                                  xlUnsigned, ...
      |                                  0);
      | 
      | 
      | % 'we' ports of 'Shared Memory' blocks
      | persistent sm_RxBuff_Radio1_we_reg; sm_RxBuff_Radio1_we_reg = xl_state(false, {xlBoolean});
      | sm_RxBuff_Radio1_we = sm_RxBuff_Radio1_we_reg;
      | opCode_sm_RxBuff_Radio1 = xl_concat(addrAck, ...
      |                                      RNWReg, ...
      |                                      bankAddr, ...
      |                                      xl_slice(linearAddr, ...
      |                                               xl_nbits(linearAddr) - 1, ...
      |                                               14) ...
      |                                     );
      | if opCode_sm_RxBuff_Radio1 == xl_concat(xfix({xlUnsigned, 4, 0}, 8), ...
      |                                          xfix({xlUnsigned, ...
      |                                                xl_nbits(linearAddr) - 14, ...
      |                                                0}, ...
      |                                                0) ...
      |                                         );
      |     sm_RxBuff_Radio1_we_reg = true;
      | else
      |     sm_RxBuff_Radio1_we_reg = false;
      | end
      | persistent sm_RxBuff_Radio2_we_reg; sm_RxBuff_Radio2_we_reg = xl_state(false, {xlBoolean});
      | sm_RxBuff_Radio2_we = sm_RxBuff_Radio2_we_reg;
      | opCode_sm_RxBuff_Radio2 = xl_concat(addrAck, ...
      |                                      RNWReg, ...
      |                                      bankAddr, ...
      |                                      xl_slice(linearAddr, ...
      |                                               xl_nbits(linearAddr) - 1, ...
      |                                               14) ...
      |                                     );
      | if opCode_sm_RxBuff_Radio2 == xl_concat(xfix({xlUnsigned, 4, 0}, 8), ...
      |                                          xfix({xlUnsigned, ...
      |                                                xl_nbits(linearAddr) - 14, ...
      |                                                0}, ...
      |                                                1) ...
      |                                         );
      |     sm_RxBuff_Radio2_we_reg = true;
      | else
      |     sm_RxBuff_Radio2_we_reg = false;
      | end
      | persistent sm_RxBuff_Radio3_we_reg; sm_RxBuff_Radio3_we_reg = xl_state(false, {xlBoolean});
      | sm_RxBuff_Radio3_we = sm_RxBuff_Radio3_we_reg;
      | opCode_sm_RxBuff_Radio3 = xl_concat(addrAck, ...
      |                                      RNWReg, ...
      |                                      bankAddr, ...
      |                                      xl_slice(linearAddr, ...
      |                                               xl_nbits(linearAddr) - 1, ...
      |                                               14) ...
      |                                     );
      | if opCode_sm_RxBuff_Radio3 == xl_concat(xfix({xlUnsigned, 4, 0}, 8), ...
      |                                          xfix({xlUnsigned, ...
      |                                                xl_nbits(linearAddr) - 14, ...
      |                                                0}, ...
      |                                                2) ...
      |                                         );
      |     sm_RxBuff_Radio3_we_reg = true;
      | else
      |     sm_RxBuff_Radio3_we_reg = false;
      | end
      | persistent sm_RxBuff_Radio4_we_reg; sm_RxBuff_Radio4_we_reg = xl_state(false, {xlBoolean});
      | sm_RxBuff_Radio4_we = sm_RxBuff_Radio4_we_reg;
      | opCode_sm_RxBuff_Radio4 = xl_concat(addrAck, ...
      |                                      RNWReg, ...
      |                                      bankAddr, ...
      |                                      xl_slice(linearAddr, ...
      |                                               xl_nbits(linearAddr) - 1, ...
      |                                               14) ...
      |                                     );
      | if opCode_sm_RxBuff_Radio4 == xl_concat(xfix({xlUnsigned, 4, 0}, 8), ...
      |                                          xfix({xlUnsigned, ...
      |                                                xl_nbits(linearAddr) - 14, ...
      |                                                0}, ...
      |                                                3) ...
      |                                         );
      |     sm_RxBuff_Radio4_we_reg = true;
      | else
      |     sm_RxBuff_Radio4_we_reg = false;
      | end
      | persistent sm_TxBuff_Radio1_we_reg; sm_TxBuff_Radio1_we_reg = xl_state(false, {xlBoolean});
      | sm_TxBuff_Radio1_we = sm_TxBuff_Radio1_we_reg;
      | opCode_sm_TxBuff_Radio1 = xl_concat(addrAck, ...
      |                                      RNWReg, ...
      |                                      bankAddr, ...
      |                                      xl_slice(linearAddr, ...
      |                                               xl_nbits(linearAddr) - 1, ...
      |                                               14) ...
      |                                     );
      | if opCode_sm_TxBuff_Radio1 == xl_concat(xfix({xlUnsigned, 4, 0}, 8), ...
      |                                          xfix({xlUnsigned, ...
      |                                                xl_nbits(linearAddr) - 14, ...
      |                                                0}, ...
      |                                                4) ...
      |                                         );
      |     sm_TxBuff_Radio1_we_reg = true;
      | else
      |     sm_TxBuff_Radio1_we_reg = false;
      | end
      | persistent sm_TxBuff_Radio2_we_reg; sm_TxBuff_Radio2_we_reg = xl_state(false, {xlBoolean});
      | sm_TxBuff_Radio2_we = sm_TxBuff_Radio2_we_reg;
      | opCode_sm_TxBuff_Radio2 = xl_concat(addrAck, ...
      |                                      RNWReg, ...
      |                                      bankAddr, ...
      |                                      xl_slice(linearAddr, ...
      |                                               xl_nbits(linearAddr) - 1, ...
      |                                               14) ...
      |                                     );
      | if opCode_sm_TxBuff_Radio2 == xl_concat(xfix({xlUnsigned, 4, 0}, 8), ...
      |                                          xfix({xlUnsigned, ...
      |                                                xl_nbits(linearAddr) - 14, ...
      |                                                0}, ...
      |                                                5) ...
      |                                         );
      |     sm_TxBuff_Radio2_we_reg = true;
      | else
      |     sm_TxBuff_Radio2_we_reg = false;
      | end
      | persistent sm_TxBuff_Radio3_we_reg; sm_TxBuff_Radio3_we_reg = xl_state(false, {xlBoolean});
      | sm_TxBuff_Radio3_we = sm_TxBuff_Radio3_we_reg;
      | opCode_sm_TxBuff_Radio3 = xl_concat(addrAck, ...
      |                                      RNWReg, ...
      |                                      bankAddr, ...
      |                                      xl_slice(linearAddr, ...
      |                                               xl_nbits(linearAddr) - 1, ...
      |                                               14) ...
      |                                     );
      | if opCode_sm_TxBuff_Radio3 == xl_concat(xfix({xlUnsigned, 4, 0}, 8), ...
      |                                          xfix({xlUnsigned, ...
      |                                                xl_nbits(linearAddr) - 14, ...
      |                                                0}, ...
      |                                                6) ...
      |                                         );
      |     sm_TxBuff_Radio3_we_reg = true;
      | else
      |     sm_TxBuff_Radio3_we_reg = false;
      | end
      | persistent sm_TxBuff_Radio4_we_reg; sm_TxBuff_Radio4_we_reg = xl_state(false, {xlBoolean});
      | sm_TxBuff_Radio4_we = sm_TxBuff_Radio4_we_reg;
      | opCode_sm_TxBuff_Radio4 = xl_concat(addrAck, ...
      |                                      RNWReg, ...
      |                                      bankAddr, ...
      |                                      xl_slice(linearAddr, ...
      |                                               xl_nbits(linearAddr) - 1, ...
      |                                               14) ...
      |                                     );
      | if opCode_sm_TxBuff_Radio4 == xl_concat(xfix({xlUnsigned, 4, 0}, 8), ...
      |                                          xfix({xlUnsigned, ...
      |                                                xl_nbits(linearAddr) - 14, ...
      |                                                0}, ...
      |                                                7) ...
      |                                         );
      |     sm_TxBuff_Radio4_we_reg = true;
      | else
      |     sm_TxBuff_Radio4_we_reg = false;
      | end
      | 
      | 
      | % 'addr' ports of 'Shared Memory' blocks
      | persistent sm_RxBuff_Radio1_addr_reg; 
      | sm_RxBuff_Radio1_addr_reg = xl_state(0, {xlUnsigned, 14, 0});
      | sm_RxBuff_Radio1_addr = sm_RxBuff_Radio1_addr_reg;
      | if addrAck == 1
      |     sm_RxBuff_Radio1_addr_reg = xl_slice(linearAddr, 14, 0);
      | else
      |     sm_RxBuff_Radio1_addr_reg = sm_RxBuff_Radio1_addr_reg;
      | end
      | persistent sm_RxBuff_Radio2_addr_reg; 
      | sm_RxBuff_Radio2_addr_reg = xl_state(0, {xlUnsigned, 14, 0});
      | sm_RxBuff_Radio2_addr = sm_RxBuff_Radio2_addr_reg;
      | if addrAck == 1
      |     sm_RxBuff_Radio2_addr_reg = xl_slice(linearAddr, 14, 0);
      | else
      |     sm_RxBuff_Radio2_addr_reg = sm_RxBuff_Radio2_addr_reg;
      | end
      | persistent sm_RxBuff_Radio3_addr_reg; 
      | sm_RxBuff_Radio3_addr_reg = xl_state(0, {xlUnsigned, 14, 0});
      | sm_RxBuff_Radio3_addr = sm_RxBuff_Radio3_addr_reg;
      | if addrAck == 1
      |     sm_RxBuff_Radio3_addr_reg = xl_slice(linearAddr, 14, 0);
      | else
      |     sm_RxBuff_Radio3_addr_reg = sm_RxBuff_Radio3_addr_reg;
      | end
      | persistent sm_RxBuff_Radio4_addr_reg; 
      | sm_RxBuff_Radio4_addr_reg = xl_state(0, {xlUnsigned, 14, 0});
      | sm_RxBuff_Radio4_addr = sm_RxBuff_Radio4_addr_reg;
      | if addrAck == 1
      |     sm_RxBuff_Radio4_addr_reg = xl_slice(linearAddr, 14, 0);
      | else
      |     sm_RxBuff_Radio4_addr_reg = sm_RxBuff_Radio4_addr_reg;
      | end
      | persistent sm_TxBuff_Radio1_addr_reg; 
      | sm_TxBuff_Radio1_addr_reg = xl_state(0, {xlUnsigned, 14, 0});
      | sm_TxBuff_Radio1_addr = sm_TxBuff_Radio1_addr_reg;
      | if addrAck == 1
      |     sm_TxBuff_Radio1_addr_reg = xl_slice(linearAddr, 14, 0);
      | else
      |     sm_TxBuff_Radio1_addr_reg = sm_TxBuff_Radio1_addr_reg;
      | end
      | persistent sm_TxBuff_Radio2_addr_reg; 
      | sm_TxBuff_Radio2_addr_reg = xl_state(0, {xlUnsigned, 14, 0});
      | sm_TxBuff_Radio2_addr = sm_TxBuff_Radio2_addr_reg;
      | if addrAck == 1
      |     sm_TxBuff_Radio2_addr_reg = xl_slice(linearAddr, 14, 0);
      | else
      |     sm_TxBuff_Radio2_addr_reg = sm_TxBuff_Radio2_addr_reg;
      | end
      | persistent sm_TxBuff_Radio3_addr_reg; 
      | sm_TxBuff_Radio3_addr_reg = xl_state(0, {xlUnsigned, 14, 0});
      | sm_TxBuff_Radio3_addr = sm_TxBuff_Radio3_addr_reg;
      | if addrAck == 1
      |     sm_TxBuff_Radio3_addr_reg = xl_slice(linearAddr, 14, 0);
      | else
      |     sm_TxBuff_Radio3_addr_reg = sm_TxBuff_Radio3_addr_reg;
      | end
      | persistent sm_TxBuff_Radio4_addr_reg; 
      | sm_TxBuff_Radio4_addr_reg = xl_state(0, {xlUnsigned, 14, 0});
      | sm_TxBuff_Radio4_addr = sm_TxBuff_Radio4_addr_reg;
      | if addrAck == 1
      |     sm_TxBuff_Radio4_addr_reg = xl_slice(linearAddr, 14, 0);
      | else
      |     sm_TxBuff_Radio4_addr_reg = sm_TxBuff_Radio4_addr_reg;
      | end
      | 
      | 
      | % 're' ports of 'From FIFO' blocks
      | 
      | 
      | % 'en' ports of 'To Register' blocks
      | if opCode == xl_concat(xfix({xlUnsigned, 4, 0}, 10), ...
      |                        xfix({xlUnsigned, xl_nbits(linearAddr), 0}, 0))
      |     sm_DebugRx1Buffers_en = true;
      | else
      |     sm_DebugRx1Buffers_en = false;
      | end
      | if opCode == xl_concat(xfix({xlUnsigned, 4, 0}, 10), ...
      |                        xfix({xlUnsigned, xl_nbits(linearAddr), 0}, 1))
      |     sm_DebugRx2Buffers_en = true;
      | else
      |     sm_DebugRx2Buffers_en = false;
      | end
      | if opCode == xl_concat(xfix({xlUnsigned, 4, 0}, 10), ...
      |                        xfix({xlUnsigned, xl_nbits(linearAddr), 0}, 2))
      |     sm_DebugRx3Buffers_en = true;
      | else
      |     sm_DebugRx3Buffers_en = false;
      | end
      | if opCode == xl_concat(xfix({xlUnsigned, 4, 0}, 10), ...
      |                        xfix({xlUnsigned, xl_nbits(linearAddr), 0}, 3))
      |     sm_DebugRx4Buffers_en = true;
      | else
      |     sm_DebugRx4Buffers_en = false;
      | end
      | if opCode == xl_concat(xfix({xlUnsigned, 4, 0}, 10), ...
      |                        xfix({xlUnsigned, xl_nbits(linearAddr), 0}, 4))
      |     sm_RADIO1RXBUFF_RXEN_en = true;
      | else
      |     sm_RADIO1RXBUFF_RXEN_en = false;
      | end
      | if opCode == xl_concat(xfix({xlUnsigned, 4, 0}, 10), ...
      |                        xfix({xlUnsigned, xl_nbits(linearAddr), 0}, 5))
      |     sm_RADIO1TXBUFF_TXEN_en = true;
      | else
      |     sm_RADIO1TXBUFF_TXEN_en = false;
      | end
      | if opCode == xl_concat(xfix({xlUnsigned, 4, 0}, 10), ...
      |                        xfix({xlUnsigned, xl_nbits(linearAddr), 0}, 6))
      |     sm_RADIO2RXBUFF_RXEN_en = true;
      | else
      |     sm_RADIO2RXBUFF_RXEN_en = false;
      | end
      | if opCode == xl_concat(xfix({xlUnsigned, 4, 0}, 10), ...
      |                        xfix({xlUnsigned, xl_nbits(linearAddr), 0}, 7))
      |     sm_RADIO2TXBUFF_TXEN_en = true;
      | else
      |     sm_RADIO2TXBUFF_TXEN_en = false;
      | end
      | if opCode == xl_concat(xfix({xlUnsigned, 4, 0}, 10), ...
      |                        xfix({xlUnsigned, xl_nbits(linearAddr), 0}, 8))
      |     sm_RADIO3RXBUFF_RXEN_en = true;
      | else
      |     sm_RADIO3RXBUFF_RXEN_en = false;
      | end
      | if opCode == xl_concat(xfix({xlUnsigned, 4, 0}, 10), ...
      |                        xfix({xlUnsigned, xl_nbits(linearAddr), 0}, 9))
      |     sm_RADIO3TXBUFF_TXEN_en = true;
      | else
      |     sm_RADIO3TXBUFF_TXEN_en = false;
      | end
      | if opCode == xl_concat(xfix({xlUnsigned, 4, 0}, 10), ...
      |                        xfix({xlUnsigned, xl_nbits(linearAddr), 0}, 10))
      |     sm_RADIO4RXBUFF_RXEN_en = true;
      | else
      |     sm_RADIO4RXBUFF_RXEN_en = false;
      | end
      | if opCode == xl_concat(xfix({xlUnsigned, 4, 0}, 10), ...
      |                        xfix({xlUnsigned, xl_nbits(linearAddr), 0}, 11))
      |     sm_RADIO4TXBUFF_TXEN_en = true;
      | else
      |     sm_RADIO4TXBUFF_TXEN_en = false;
      | end
      | if opCode == xl_concat(xfix({xlUnsigned, 4, 0}, 10), ...
      |                        xfix({xlUnsigned, xl_nbits(linearAddr), 0}, 12))
      |     sm_StartCapture_en = true;
      | else
      |     sm_StartCapture_en = false;
      | end
      | if opCode == xl_concat(xfix({xlUnsigned, 4, 0}, 10), ...
      |                        xfix({xlUnsigned, xl_nbits(linearAddr), 0}, 13))
      |     sm_StartTx_en = true;
      | else
      |     sm_StartTx_en = false;
      | end
      | if opCode == xl_concat(xfix({xlUnsigned, 4, 0}, 10), ...
      |                        xfix({xlUnsigned, xl_nbits(linearAddr), 0}, 14))
      |     sm_StopTx_en = true;
      | else
      |     sm_StopTx_en = false;
      | end
      | if opCode == xl_concat(xfix({xlUnsigned, 4, 0}, 10), ...
      |                        xfix({xlUnsigned, xl_nbits(linearAddr), 0}, 15))
      |     sm_TransMode_en = true;
      | else
      |     sm_TransMode_en = false;
      | end
      | if opCode == xl_concat(xfix({xlUnsigned, 4, 0}, 10), ...
      |                        xfix({xlUnsigned, xl_nbits(linearAddr), 0}, 16))
      |     sm_TxDelay_en = true;
      | else
      |     sm_TxDelay_en = false;
      | end
      | if opCode == xl_concat(xfix({xlUnsigned, 4, 0}, 10), ...
      |                        xfix({xlUnsigned, xl_nbits(linearAddr), 0}, 17))
      |     sm_TxLength_en = true;
      | else
      |     sm_TxLength_en = false;
      | end
      | 
      | 
      | % 'din' ports of 'To FIFO' blocks
      | 
      | 
      | % 'we' ports of 'To FIFO' blocks
      | 
      | 
      | % 'din' ports of 'To Register' blocks
      | sm_DebugRx1Buffers_din = xl_force(xl_slice(wrDBus, 1 - 1, 0), ...
      |                                  xlUnsigned, ...
      |                                  0);
      | sm_DebugRx2Buffers_din = xl_force(xl_slice(wrDBus, 1 - 1, 0), ...
      |                                  xlUnsigned, ...
      |                                  0);
      | sm_DebugRx3Buffers_din = xl_force(xl_slice(wrDBus, 1 - 1, 0), ...
      |                                  xlUnsigned, ...
      |                                  0);
      | sm_DebugRx4Buffers_din = xl_force(xl_slice(wrDBus, 1 - 1, 0), ...
      |                                  xlUnsigned, ...
      |                                  0);
      | sm_RADIO1RXBUFF_RXEN_din = xl_force(xl_slice(wrDBus, 1 - 1, 0), ...
      |                                  xlUnsigned, ...
      |                                  0);
      | sm_RADIO1TXBUFF_TXEN_din = xl_force(xl_slice(wrDBus, 1 - 1, 0), ...
      |                                  xlUnsigned, ...
      |                                  0);
      | sm_RADIO2RXBUFF_RXEN_din = xl_force(xl_slice(wrDBus, 1 - 1, 0), ...
      |                                  xlUnsigned, ...
      |                                  0);
      | sm_RADIO2TXBUFF_TXEN_din = xl_force(xl_slice(wrDBus, 1 - 1, 0), ...
      |                                  xlUnsigned, ...
      |                                  0);
      | sm_RADIO3RXBUFF_RXEN_din = xl_force(xl_slice(wrDBus, 1 - 1, 0), ...
      |                                  xlUnsigned, ...
      |                                  0);
      | sm_RADIO3TXBUFF_TXEN_din = xl_force(xl_slice(wrDBus, 1 - 1, 0), ...
      |                                  xlUnsigned, ...
      |                                  0);
      | sm_RADIO4RXBUFF_RXEN_din = xl_force(xl_slice(wrDBus, 1 - 1, 0), ...
      |                                  xlUnsigned, ...
      |                                  0);
      | sm_RADIO4TXBUFF_TXEN_din = xl_force(xl_slice(wrDBus, 1 - 1, 0), ...
      |                                  xlUnsigned, ...
      |                                  0);
      | sm_StartCapture_din = xl_force(xl_slice(wrDBus, 1 - 1, 0), ...
      |                                  xlUnsigned, ...
      |                                  0);
      | sm_StartTx_din = xl_force(xl_slice(wrDBus, 1 - 1, 0), ...
      |                                  xlUnsigned, ...
      |                                  0);
      | sm_StopTx_din = xl_force(xl_slice(wrDBus, 1 - 1, 0), ...
      |                                  xlUnsigned, ...
      |                                  0);
      | sm_TransMode_din = xl_force(xl_slice(wrDBus, 1 - 1, 0), ...
      |                                  xlUnsigned, ...
      |                                  0);
      | sm_TxDelay_din = xl_force(xl_slice(wrDBus, 14 - 1, 0), ...
      |                                  xlUnsigned, ...
      |                                  0);
      | sm_TxLength_din = xl_force(xl_slice(wrDBus, 14 - 1, 0), ...
      |                                  xlUnsigned, ...
      |                                  0);
      | 
      | 
      | persistent read_bank_out_reg; read_bank_out_reg = xl_state(0, {xlUnsigned, 32, 0});
      | read_bank_out = read_bank_out_reg;
      | 
      | persistent bankAddr_reg; bankAddr_reg = xl_state(0, bankAddr);
      | 
      | if bankAddr_reg == 0
      |     % Bank 0: Shared Memories
      |     read_bank_out_reg = ram_bank_out;
      | elseif bankAddr_reg == 1
      |     % Bank 1: From/To FIFOs
      |     read_bank_out_reg =  0;
      | elseif bankAddr_reg == 2
      |     % Bank 2: From/To Registers
      |     read_bank_out_reg = reg_bank_out;
      | elseif bankAddr_reg == 3
      |     % Bank 3: Configuration Registers
      |     read_bank_out_reg = 0;
      | end
      | 
      | bankAddr_reg = bankAddr;
      settings: block_version=10.1.3
  sg_plb_addrpref : xbsIndex_r4/Gateway In  arith_type=Unsigned  n_bits=11  bin_pt=0  quantization="Round  (unbiased: +/- Inf)"  overflow=Saturate  period=xlGetSimulinkPeriod(gcb)  dbl_ovrd=off  timing_constraint=None  locs_specified=off  LOCs={}  block_type=gatewayin
      settings: infoedit="Gateway in block.  Converts inputs of type Simulink integer, double and fixed point to  Xilinx fixed point type.<P><P>Hardware notes:  In hardware these blocks become top level input ports."  sginterface={'Xilinx'=>{'jtaghwcosim'=>{'non_memory_mapped_port'=>'sg_plb_addrpref'}},'iopad'=>{'constraint'=>'#'}}  block_version=10.1.3
  wires:
  plb_decode/2 -> plb_memmap/5, Sl_addrAck/1  "Sl_addrAck"
  plb_decode/4 -> Sl_wrDAck/1, Sl_wrComp/1  "Sl_wrDAck"
  plb_memmap/61 -> Shared Memory7/3  "TxBuff_Radio4_we"
  plb_memmap/60 -> Shared Memory7/2  "TxBuff_Radio4_din"
  plb_memmap/59 -> Shared Memory7/1  "TxBuff_Radio4_addr"
  plb_memmap/58 -> Shared Memory6/3  "TxBuff_Radio3_we"
  plb_memmap/57 -> Shared Memory6/2  "TxBuff_Radio3_din"
  plb_memmap/56 -> Shared Memory6/1  "TxBuff_Radio3_addr"
  plb_memmap/55 -> Shared Memory5/3  "TxBuff_Radio2_we"
  plb_memmap/54 -> Shared Memory5/2  "TxBuff_Radio2_din"
  plb_memmap/53 -> Shared Memory5/1  "TxBuff_Radio2_addr"
  plb_memmap/52 -> Shared Memory4/3  "TxBuff_Radio1_we"
  plb_memmap/51 -> Shared Memory4/2  "TxBuff_Radio1_din"
  plb_memmap/50 -> Shared Memory4/1  "TxBuff_Radio1_addr"
  plb_memmap/49 -> Shared Memory3/3  "RxBuff_Radio4_we"
  plb_memmap/48 -> Shared Memory3/2  "RxBuff_Radio4_din"
  plb_memmap/47 -> Shared Memory3/1  "RxBuff_Radio4_addr"
  plb_memmap/46 -> Shared Memory2/3  "RxBuff_Radio3_we"
  plb_memmap/45 -> Shared Memory2/2  "RxBuff_Radio3_din"
  plb_memmap/44 -> Shared Memory2/1  "RxBuff_Radio3_addr"
  plb_memmap/43 -> Shared Memory1/3  "RxBuff_Radio2_we"
  plb_memmap/42 -> Shared Memory1/2  "RxBuff_Radio2_din"
  plb_memmap/41 -> Shared Memory1/1  "RxBuff_Radio2_addr"
  plb_memmap/40 -> Shared Memory/3  "RxBuff_Radio1_we"
  plb_memmap/39 -> Shared Memory/2  "RxBuff_Radio1_din"
  plb_memmap/38 -> Shared Memory/1  "RxBuff_Radio1_addr"
  plb_memmap/37 -> To Register17/2  "TxLength_en"
  plb_memmap/36 -> To Register17/1  "TxLength_din"
  plb_memmap/35 -> To Register16/2  "TxDelay_en"
  plb_memmap/34 -> To Register16/1  "TxDelay_din"
  plb_memmap/33 -> To Register15/2  "TransMode_en"
  plb_memmap/32 -> To Register15/1  "TransMode_din"
  plb_memmap/31 -> To Register14/2  "StopTx_en"
  plb_memmap/30 -> To Register14/1  "StopTx_din"
  plb_memmap/29 -> To Register13/2  "StartTx_en"
  plb_memmap/28 -> To Register13/1  "StartTx_din"
  plb_memmap/27 -> To Register12/2  "StartCapture_en"
  plb_memmap/26 -> To Register12/1  "StartCapture_din"
  plb_memmap/25 -> To Register11/2  "RADIO4TXBUFF_TXEN_en"
  plb_memmap/24 -> To Register11/1  "RADIO4TXBUFF_TXEN_din"
  plb_memmap/23 -> To Register10/2  "RADIO4RXBUFF_RXEN_en"
  plb_memmap/22 -> To Register10/1  "RADIO4RXBUFF_RXEN_din"
  plb_memmap/21 -> To Register9/2  "RADIO3TXBUFF_TXEN_en"
  plb_memmap/20 -> To Register9/1  "RADIO3TXBUFF_TXEN_din"
  plb_memmap/19 -> To Register8/2  "RADIO3RXBUFF_RXEN_en"
  plb_memmap/18 -> To Register8/1  "RADIO3RXBUFF_RXEN_din"
  plb_memmap/17 -> To Register7/2  "RADIO2TXBUFF_TXEN_en"
  plb_memmap/16 -> To Register7/1  "RADIO2TXBUFF_TXEN_din"
  plb_memmap/15 -> To Register6/2  "RADIO2RXBUFF_RXEN_en"
  plb_memmap/14 -> To Register6/1  "RADIO2RXBUFF_RXEN_din"
  plb_memmap/13 -> To Register5/2  "RADIO1TXBUFF_TXEN_en"
  plb_memmap/12 -> To Register5/1  "RADIO1TXBUFF_TXEN_din"
  plb_memmap/11 -> To Register4/2  "RADIO1RXBUFF_RXEN_en"
  plb_memmap/10 -> To Register4/1  "RADIO1RXBUFF_RXEN_din"
  plb_memmap/9 -> To Register3/2  "DebugRx4Buffers_en"
  plb_memmap/8 -> To Register3/1  "DebugRx4Buffers_din"
  plb_memmap/7 -> To Register2/2  "DebugRx3Buffers_en"
  plb_memmap/6 -> To Register2/1  "DebugRx3Buffers_din"
  plb_memmap/5 -> To Register1/2  "DebugRx2Buffers_en"
  plb_memmap/4 -> To Register1/1  "DebugRx2Buffers_din"
  plb_memmap/3 -> To Register/2  "DebugRx1Buffers_en"
  plb_memmap/2 -> To Register/1  "DebugRx1Buffers_din"
  plb_memmap/1 -> plb_decode/6  "rdData"
  Shared Memory7/1 -> plb_memmap/32  "TxBuff_Radio4_dout"
  Shared Memory6/1 -> plb_memmap/31  "TxBuff_Radio3_dout"
  Shared Memory5/1 -> plb_memmap/30  "TxBuff_Radio2_dout"
  Shared Memory4/1 -> plb_memmap/29  "TxBuff_Radio1_dout"
  Shared Memory3/1 -> plb_memmap/28  "RxBuff_Radio4_dout"
  Shared Memory2/1 -> plb_memmap/27  "RxBuff_Radio3_dout"
  Shared Memory1/1 -> plb_memmap/26  "RxBuff_Radio2_dout"
  Shared Memory/1 -> plb_memmap/25  "RxBuff_Radio1_dout"
  To Register17/1 -> plb_memmap/24  "TxLength_dout"
  To Register16/1 -> plb_memmap/23  "TxDelay_dout"
  To Register15/1 -> plb_memmap/22  "TransMode_dout"
  To Register14/1 -> plb_memmap/21  "StopTx_dout"
  To Register13/1 -> plb_memmap/20  "StartTx_dout"
  To Register12/1 -> plb_memmap/19  "StartCapture_dout"
  To Register11/1 -> plb_memmap/18  "RADIO4TXBUFF_TXEN_dout"
  To Register10/1 -> plb_memmap/17  "RADIO4RXBUFF_RXEN_dout"
  To Register9/1 -> plb_memmap/16  "RADIO3TXBUFF_TXEN_dout"
  To Register8/1 -> plb_memmap/15  "RADIO3RXBUFF_RXEN_dout"
  To Register7/1 -> plb_memmap/14  "RADIO2TXBUFF_TXEN_dout"
  To Register6/1 -> plb_memmap/13  "RADIO2RXBUFF_RXEN_dout"
  To Register5/1 -> plb_memmap/12  "RADIO1TXBUFF_TXEN_dout"
  To Register4/1 -> plb_memmap/11  "RADIO1RXBUFF_RXEN_dout"
  To Register3/1 -> plb_memmap/10  "DebugRx4Buffers_dout"
  To Register2/1 -> plb_memmap/9  "DebugRx3Buffers_dout"
  To Register1/1 -> plb_memmap/8  "DebugRx2Buffers_dout"
  To Register/1 -> plb_memmap/7  "DebugRx1Buffers_dout"
  From Register/1 -> plb_memmap/6  "CaptureDone_dout"
  plb_decode/6 -> plb_memmap/4  "RNWReg"
  plb_decode/9 -> plb_memmap/3  "linearAddr"
  plb_decode/5 -> plb_memmap/2  "bankAddr"
  plb_decode/1 -> plb_memmap/1  "wrDBusReg"
  plb_decode/8 -> Sl_rdDBus/1  "Sl_rdDBus"
  plb_decode/7 -> Sl_rdDAck/1  "Sl_rdDAck"
  plb_decode/3 -> Sl_rdComp/1  "Sl_rdComp"
  sg_plb_addrpref/1 -> plb_decode/7  "addrPref"
  PLB_wrDBus/1 -> plb_decode/5  "PLB_wrDBus"
  PLB_RNW/1 -> plb_decode/4  "PLB_RNW"
  PLB_PAValid/1 -> plb_decode/3  "PLB_PAValid"
  PLB_ABus/1 -> plb_decode/2  "PLB_ABus"
  SPLB_Rst/1 -> plb_decode/1  "SPLB_Rst"
  Constant6/1 -> sg_plb_addrpref/1
  Constant5/1 -> Sl_wait/1  "Sl_wait"
  Constant4/1 -> PLB_wrDBus/1
  Constant3/1 -> PLB_RNW/1
  Constant2/1 -> PLB_PAValid/1
  Constant1/1 -> PLB_ABus/1
  Constant/1 -> SPLB_Rst/1
  Sl_wrComp/1 -> Terminator6/1
  Sl_wrDAck/1 -> Terminator5/1
  Sl_wait/1 -> Terminator4/1
  Sl_rdDBus/1 -> Terminator3/1
  Sl_rdDAck/1 -> Terminator2/1
  Sl_rdComp/1 -> Terminator1/1
  Sl_addrAck/1 -> Terminator/1
